simulink model "test_ffts"  (Simulink 6.2)
settings: Solver=ode45  StartTime=0.0  StopTime=300  RelTol=1e-3
undefined symbols (not defined in the file or in its folder): now
libraries: xbsIndex_r3 x1135, fft_library x1, simulink x1
(part 1 of 15)
settings Model: LastModifiedBy=mdexter
settings DebuggingCC: SolverPrmCheckMsg=warning

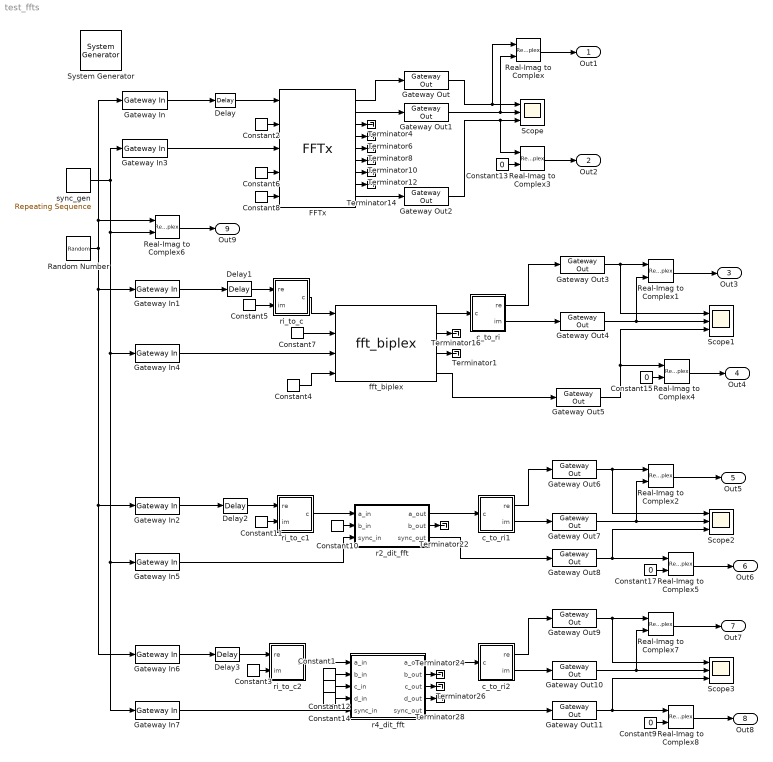
== system test_ffts ==
  " System Generator" : xbsIndex_r3/ System Generator  Tag=genX  xilinxfamily=Virtex2  part=xc2v1000  speed=-4  package=bg575  synthesis_tool=XST  directory=./netlist  testbench=off  simulink_period=1  sysclk_period=100  incr_netlist=off  trim_vbits=Everywhere in SubSystem  dbl_ovrd=According to Block Masks  core_generation=According to Block Masks  run_coregen=off  deprecated_control=off  eval_field=0
      settings: AttributesFormatString=System\nGenerator
  Constant{1,10,12,14} (4 alike) : xbsIndex_r3/Constant  const=0  equ=P=C  arith_type=Unsigned  n_bits=16  bin_pt=0  opselect=C  inp2=PCIN>>17  opr=+  inp1=P  carry=CIN  iostate=0  explicit_period=on  period=1  dbl_ovrd=off
  Constant11 : xbsIndex_r3/Constant  const=0  equ=P=C  arith_type=Unsigned  n_bits=8  bin_pt=7  opselect=C  inp2=PCIN>>17  opr=+  inp1=P  carry=CIN  iostate=0  explicit_period=on  period=1  dbl_ovrd=off
  Constant{9,13,15,17} (4 alike) : Constant  Value=0
  Constant2 : xbsIndex_r3/Constant  const=0  equ=P=C  arith_type="Signed  (2's comp)"  n_bits=8  bin_pt=7  opselect=C  inp2=PCIN>>17  opr=+  inp1=P  carry=CIN  iostate=0  explicit_period=on  period=1  dbl_ovrd=off
  Constant3 : xbsIndex_r3/Constant  const=0  equ=P=C  arith_type=Unsigned  n_bits=8  bin_pt=7  opselect=C  inp2=PCIN>>17  opr=+  inp1=P  carry=CIN  iostate=0  explicit_period=on  period=1  dbl_ovrd=off
  Constant4 : xbsIndex_r3/Constant  const=0  equ=P=C  arith_type=Unsigned  n_bits=6  bin_pt=0  opselect=C  inp2=PCIN>>17  opr=+  inp1=P  carry=CIN  iostate=0  explicit_period=on  period=1  dbl_ovrd=off
  Constant5 : xbsIndex_r3/Constant  const=0  equ=P=C  arith_type=Unsigned  n_bits=18  bin_pt=0  opselect=C  inp2=PCIN>>17  opr=+  inp1=P  carry=CIN  iostate=0  explicit_period=on  period=1  dbl_ovrd=off
  Constant6 : xbsIndex_r3/Constant  const=1  equ=P=C  arith_type=Boolean  n_bits=1  bin_pt=0  opselect=C  inp2=PCIN>>17  opr=+  inp1=P  carry=CIN  iostate=0  explicit_period=on  period=1  dbl_ovrd=off
  Constant7 : xbsIndex_r3/Constant  const=0  equ=P=C  arith_type=Unsigned  n_bits=36  bin_pt=0  opselect=C  inp2=PCIN>>17  opr=+  inp1=P  carry=CIN  iostate=0  explicit_period=on  period=1  dbl_ovrd=off
  Constant8 : xbsIndex_r3/Constant  const=1  equ=P=C  arith_type=Boolean  n_bits=1  bin_pt=0  opselect=C  inp2=PCIN>>17  opr=+  inp1=P  carry=CIN  iostate=0  explicit_period=on  period=1  dbl_ovrd=off
  Delay : xbsIndex_r3/Delay  latency=4  reg_retiming=off  explicit_period=off  period=1  en=off  accept_only_valid=off  init_zero=on  dbl_ovrd=off  show_param=off
      settings: xl_area=[0, 0, 0, 0, 0, 0, 0]
  Delay1 : xbsIndex_r3/Delay  latency=1  reg_retiming=off  explicit_period=off  period=1  en=off  accept_only_valid=off  init_zero=on  dbl_ovrd=off  show_param=off
      settings: xl_area=[0, 0, 0, 0, 0, 0, 0]
  Delay2 : xbsIndex_r3/Delay  latency=1  reg_retiming=off  explicit_period=off  period=1  en=off  accept_only_valid=off  init_zero=on  dbl_ovrd=off  show_param=off
      settings: xl_area=[0, 0, 0, 0, 0, 0, 0]
  Delay3 : xbsIndex_r3/Delay  latency=1  reg_retiming=off  explicit_period=off  period=1  en=off  accept_only_valid=off  init_zero=on  dbl_ovrd=off  show_param=off
      settings: xl_area=[0, 0, 0, 0, 0, 0, 0]
  FFTx : xbsIndex_r3/FFTx  arch=Pipelined Streaming I/O  npts=64  scaling=Unscaled  rounding=Convergent Rounding  tf_width=8  op_order=Natural Order  twiddle_mem_type=Block RAM  data_mem_type=Block RAM  num_bram_stages=0  explicit_period=off  period=-1  use_dsp48=off  en_n=off  has_ovflo=off  rst=off  en=off  dbl_ovrd=off  show_param=on  gen_core=off
      settings: xl_area=[0, 0, 0, 0, 0, 0, 0]
  Gateway In : xbsIndex_r3/Gateway In  arith_type="Signed  (2's comp)"  n_bits=8  bin_pt=7  quantization="Round  (unbiased: +/- Inf)"  overflow=Wrap  period=1  timing_constraint=None  locs_specified=off  LOCs={}  needs_fixed_name=off  dbl_ovrd=off  show_param=off
      settings: xl_area=[0, 0, 0, 0, 0, 0, 0]
  Gateway In1 : xbsIndex_r3/Gateway In  arith_type="Signed  (2's comp)"  n_bits=18  bin_pt=14  quantization="Round  (unbiased: +/- Inf)"  overflow=Wrap  period=1  timing_constraint=None  locs_specified=off  LOCs={}  needs_fixed_name=off  dbl_ovrd=off  show_param=off
      settings: xl_area=[0, 0, 0, 0, 0, 0, 0]
  Gateway In2 : xbsIndex_r3/Gateway In  arith_type="Signed  (2's comp)"  n_bits=8  bin_pt=7  quantization="Round  (unbiased: +/- Inf)"  overflow=Wrap  period=1  timing_constraint=None  locs_specified=off  LOCs={}  needs_fixed_name=off  dbl_ovrd=off  show_param=off
      settings: xl_area=[0, 0, 0, 0, 0, 0, 0]
  Gateway In{3..5,7} (4 alike) : xbsIndex_r3/Gateway In  arith_type=Boolean  n_bits=8  bin_pt=7  quantization=Truncate  overflow=Wrap  period=1  timing_constraint=None  locs_specified=off  LOCs={}  needs_fixed_name=off  dbl_ovrd=off  show_param=off
      settings: xl_area=[0, 0, 0, 0, 0, 0, 0]
  Gateway In6 : xbsIndex_r3/Gateway In  arith_type="Signed  (2's comp)"  n_bits=8  bin_pt=7  quantization="Round  (unbiased: +/- Inf)"  overflow=Wrap  period=1  timing_constraint=None  locs_specified=off  LOCs={}  needs_fixed_name=off  dbl_ovrd=off  show_param=off
      settings: xl_area=[0, 0, 0, 0, 0, 0, 0]
  Gateway Out{,1..11} (12 alike) : xbsIndex_r3/Gateway Out  output_type=Double  nbits=8  bin_pt=6  arith_type=Boolean  quantization=Truncate  overflow=Wrap  hdl_port=on  timing_constraint=None  locs_specified=off  LOCs={}  needs_fixed_name=off  show_param=off
      settings: xl_area=[0, 0, 0, 0, 0, 0, 0]
  Random Number : RandomNumber  Variance=.3^2  Seed=floor(100*(now-floor(now)))  SampleTime=1
  Real-Imag to Complex{,1..8} (9 alike) : RealImagToComplex
  Scope{,1..3} (4 alike) : Scope  NumInputPorts=3
      Scope settings: YMin=-5~-5~-5  YMax=5~5~5
      Scope1 settings: YMin=-5~-5~-5  YMax=5~5~5
      Scope2 settings: YMin=-5~-5~-5  YMax=5~5~5  SaveName=ScopeData2
      Scope3 settings: YMin=-5~-5~-5  YMax=5~5~5  SaveName=ScopeData3
  Terminator{1,4,6,8,10,12,14,16,22,24,26,28} (12 alike) : Terminator
  c_to_ri : Subsystem  mask(Complex to Real-Imag){n_bits=18, bin_pt=14}
      mask prompts: n_bits "Bit Width"; bin_pt "Binary Point"
      mask help: Outputs real and imaginary components of a complex input.
      mask init:
      | c_to_ri_init(gcb,n_bits,bin_pt);
      settings: AttributesFormatString=%<n_bits>_%<bin_pt> r/i
      mask Help:
      | <pre>
      | Description::
      | 
      | Outputs real and imaginary components of a complex input.
      | Useful for simplifying interconnects.
      | See also: Real-Imag to Complex (ri_to_c)
      | 
      | Mask Parameters::
      | 
      | Bit Width (n_bits): Specifies the width of the real/imaginary components.
      | Assumed equal for both components.
      | 
      | Binary Point (bin_pt): Specifies the binary point location in the real/imaginary components.
      | Assumed equal for both components.
      | </pre>
  c_to_ri1 : Subsystem  mask(Complex to Real-Imag){n_bits=14, bin_pt=7}
      mask prompts: n_bits "Bit Width"; bin_pt "Binary Point"
      mask help: Outputs real and imaginary components of a complex input.
      mask init:
      | c_to_ri_init(gcb,n_bits,bin_pt);
      settings: AttributesFormatString=14_7 r/i
      mask Help:
      | <pre>
      | Description::
      | 
      | Outputs real and imaginary components of a complex input.
      | Useful for simplifying interconnects.
      | See also: Real-Imag to Complex (ri_to_c)
      | 
      | Mask Parameters::
      | 
      | Bit Width (n_bits): Specifies the width of the real/imaginary components.
      | Assumed equal for both components.
      | 
      | Binary Point (bin_pt): Specifies the binary point location in the real/imaginary components.
      | Assumed equal for both components.
      | </pre>
  c_to_ri2 : Subsystem  mask(Complex to Real-Imag){n_bits=14, bin_pt=7}
      mask prompts: n_bits "Bit Width"; bin_pt "Binary Point"
      mask help: Outputs real and imaginary components of a complex input.
      mask init:
      | c_to_ri_init(gcb,n_bits,bin_pt);
      settings: AttributesFormatString=%<n_bits>_%<bin_pt> r/i
      mask Help:
      | <pre>
      | Description::
      | 
      | Outputs real and imaginary components of a complex input.
      | Useful for simplifying interconnects.
      | See also: Real-Imag to Complex (ri_to_c)
      | 
      | Mask Parameters::
      | 
      | Bit Width (n_bits): Specifies the width of the real/imaginary components.
      | Assumed equal for both components.
      | 
      | Binary Point (bin_pt): Specifies the binary point location in the real/imaginary components.
      | Assumed equal for both components.
      | </pre>
  fft_biplex : fft_library/fft_biplex  FFTSize=6  BitWidth=18  quantization="Round  (unbiased: Even Values)"  overflow=Saturate  add_latency=1  mult_latency=3  bram_latency=1
      link override biplex_core/fft_stage_1/sync_delay_x/Constant: equ=P=C
      link override biplex_core/fft_stage_1/sync_delay_x/Constant1: equ=P=C
      link override biplex_core/fft_stage_1/sync_delay_x/Constant2: equ=P=C
      link override biplex_core/fft_stage_1/sync_delay_x/Constant3: equ=P=C
      link override biplex_core/fft_stage_2/sync_delay_x/Constant: equ=P=C
      link override biplex_core/fft_stage_2/sync_delay_x/Constant1: equ=P=C
      link override biplex_core/fft_stage_2/sync_delay_x/Constant2: equ=P=C
      link override biplex_core/fft_stage_2/sync_delay_x/Constant3: equ=P=C
      link override biplex_core/fft_stage_3/sync_delay_x/Constant: equ=P=C
      link override biplex_core/fft_stage_3/sync_delay_x/Constant1: equ=P=C
      link override biplex_core/fft_stage_3/sync_delay_x/Constant2: equ=P=C
      link override biplex_core/fft_stage_3/sync_delay_x/Constant3: equ=P=C
      link override biplex_core/fft_stage_4/sync_delay_x/Constant: equ=P=C
      link override biplex_core/fft_stage_4/sync_delay_x/Constant1: equ=P=C
      link override biplex_core/fft_stage_4/sync_delay_x/Constant2: equ=P=C
      link override biplex_core/fft_stage_4/sync_delay_x/Constant3: equ=P=C
      link override biplex_core/fft_stage_5/sync_delay_x/Constant: equ=P=C
      link override biplex_core/fft_stage_5/sync_delay_x/Constant1: equ=P=C
      link override biplex_core/fft_stage_5/sync_delay_x/Constant2: equ=P=C
      link override biplex_core/fft_stage_5/sync_delay_x/Constant3: equ=P=C
      link override biplex_core/fft_stage_6/sync_delay_x/Constant: equ=P=C
      link override biplex_core/fft_stage_6/sync_delay_x/Constant1: equ=P=C
      link override biplex_core/fft_stage_6/sync_delay_x/Constant2: equ=P=C
      link override biplex_core/fft_stage_6/sync_delay_x/Constant3: equ=P=C
      link override biplex_cplx_unscrambler/delay_bram1/Constant2: equ=P=C
      link override biplex_cplx_unscrambler/reorder/Constant: equ=P=C
      link override biplex_cplx_unscrambler/reorder/sync_delay/Constant: equ=P=C
      link override biplex_cplx_unscrambler/reorder/sync_delay/Constant1: equ=P=C
      link override biplex_cplx_unscrambler/reorder/sync_delay/Constant2: equ=P=C
      link override biplex_cplx_unscrambler/reorder/sync_delay/Constant3: equ=P=C
      link override biplex_cplx_unscrambler/reorder1/Constant: equ=P=C
      link override biplex_cplx_unscrambler/reorder1/sync_delay/Constant: equ=P=C
      link override biplex_cplx_unscrambler/reorder1/sync_delay/Constant1: equ=P=C
      link override biplex_cplx_unscrambler/reorder1/sync_delay/Constant2: equ=P=C
      link override biplex_cplx_unscrambler/reorder1/sync_delay/Constant3: equ=P=C
      link override biplex_cplx_unscrambler/sync_delay/Constant: equ=P=C
      link override biplex_cplx_unscrambler/sync_delay/Constant1: equ=P=C
      link override biplex_cplx_unscrambler/sync_delay/Constant2: equ=P=C
      link override biplex_cplx_unscrambler/sync_delay/Constant3: equ=P=C
  r2_dit_fft : Subsystem  AncestorBlock=newfft_library/FFT/r2_dit_fft  mask(Biplex Radix-2 DIT FFT){n_stages=6, n_bits=8, bin_pt=7, shifts=[0], commutator_bram=0, twiddle_bram=0, n_bits_w=9, mult_latency=3, add_latency=1, commute_output=Yes (BRAM), output_order=Normal, show_sbo=on, munge_submasks=DumbDown}
      mask prompts: n_stages "Total Stages"; n_bits "Number of Bits In"; bin_pt "Binary Point In"; shifts "Shifting Schedule"; commutator_bram "Number of Stages Using BRAM for Biplex Commutators (i.e. delays)"; twiddle_bram "Number of Stages Using BRAM for Twiddle Coefficients"; n_bits_w "Twiddle Coefficient Bitwidth"; mult_latency "Multiplier Latency"; add_latency "Adder Latency"; commute_output "Commute Output"; output_order "Output Order"; show_sbo "Show Sub-Block Options"; munge_submasks "Sub-Block Masks"
      mask help: A biplex radix-2 decimation-in-time Fast Fourier Transform.
      mask init:
      | tic
      | r2_dit_fft_init(gcb, ...
      |   n_stages, ...
      |   n_bits, ...
      |   bin_pt, ...
      |   shifts, ...
      |   commutator_bram, ...
      |   twiddle_bram, ...
      |   n_bits_w, ...
      |   mult_latency, ...
      |   add_latency, ...
      |   commute_output, ...
      |   output_order, ...
      |   lower(get_param(gcb,'munge_submasks')) );
      | disp('r2_dit_fft initialization complete.');
      | toc
      settings: AttributesFormatString=|
      | 64 points
      | 8_7 r/i in
      | 9_7 twiddles
      mask Help:
      | <pre>
      | Description::
      | 
      | A biplex radix-2 decimation-in-time Fast Fourier Transform.
      | 
      | The two inputs to the biplex FFT are independent complex signals (e.g. A and B).
      | 
      | Without an output commutator, the two outputs of the FFT are commuted such that the a_out
      | signal is really the "lower" half of A's transform followed by the "lower" half of B's
      | transform and b_out is really the "upper" half of A's transform followed by the "upper"
      | half of B's transform.
      | 
      | If it is desired to have the two halves of A's transform follow each other on the same path
      | and the two halves of B's transform follow each other on the same path, then be sure to
      | check the "Output Commutator" checkbox.  This will result in the "lower" half of A (or B)
      | followed by the "upper" half of A (or B).  Including the output commutator uses additional
      | resources.
      | 
      | If the "Normal" Ouput Order option is chosen, the output will be in normal order (though still in
      | commuted halves if no output commutator is used).  If the "Bit Reversed" Output Order" option is
      | selected, the output halves (either commuted or not) will each be in bit reversed order
      | (i.e. each half of each transform will be in bit reversed output order).   Normal output is easier
      | for humans to work with (especially for testing), but it uses additional resources.  Bit reversed
      | output is the implementation's inhernet output order so that option uses no additional resources.
      | 
      | The number of bits for each real and imaginary component grows by two through each stage.
      | If a stage's input bit width is 17 or less, three embedded multipliers will be used per complex multiply.
      | If a stage's input bit width is 18, four embedded multipliers will be used per complex multiply.
      | If a stage's input bit width exceeds 18, then substantially more embedded multipliers will be used
      | per complex multiply.  Enabling "shifting" in some (or all) stages can limit the bit growth
      | to prevent this.  See the Shifting Schedule parameter for more info.
      | 
      | Mask Parameters::
      | 
      | Total Stages (n_stages):  The number of total stages in the FFT.
      | The FFT will have 2^n_stages points.
      | 
      | Number of Bits In (n_bits): Specifies the width of the real/imaginary components of ports
      | a_in and b_in.  Assumed equal for both components.  The output bit width will be
      | n_bits+n_stages (assuming sum(shifts)==0).
      | 
      | Binary Point In (bin_pt): Specifies the binary point position of the real/imaginary
      | components of ports a_in and b_in.  Assumed equal for both components.
      | 
      | Shifting Schedule (shifts): A vector specifying how many bits to shift by at each stage.
      | Missing values are assumed to be zero; extra values are ignored.
      | 
      | Number of Stages Using BRAM for Biplex Commutators (commutator_bram): Number of stages
      | that will use BRAM for commutator memory.  Remaining stages will use SLR16 elements (slices).
      | 
      | Number of Stages Using BRAM for Twiddle Coefficients (twiddle_bram): Number of stages that
      | will use BRAM for twiddle coeeficient storage.  Remaining stages will use distributed memory
      | (slices).
      | 
      | Twiddle Coefficient Bitwidth (n_bits_w): Specifies the width of the real/imaginary
      | components of the twiddle coefficients.  Assumed equal for both components.
      | 
      | Multiplier Latency (mult_latency): Latency to use for the underlying real multipliers.
      | 
      | Adder Latency (add_latency): Latency to use for the underlying real adders.
      | 
      | Commute Output (commute_output): Popup options for an output commutator.  See decription
      | above for details on the output commutator.  Choices are:
      |     "No" - No output commutator
      |     "Yes (SLR16)" - Include output commutator using SLR16 elements
      |     "Yes (BRAM)" - Include output commutator using BRAM
      | 
      | Output Order (output_order): Popup options for selecting the output order.  See description
      | above for details on the output order.  Choices are:
      |     "Bit Reversed" - Output each half of each transform in bit reversed order.
      |     "Normal" - Output each half of each transform in normal order.
      | </pre>
      mask StyleString: edit,edit,edit,edit,edit,edit,edit,edit,edit,popup(No|Yes (SLR16)|Yes (BRAM)),popup(Bit Reversed|Normal),checkbox,popup(Keep|DumbDown|Unmask)
      mask CallbackString:
      | |||||||||||mvs=get_param(gcb,'MaskVisibilityString');
      | if strcmp(get_param(gcb,'show_sbo'),'on')
      |   onoff='on';
      | else
      |   onoff='off';
      | end
      | mvs=regexprep(mvs,'o[nf]*$',onoff);
      | set_param(gcb,'MaskVisibilityString',mvs);
      | |mvs=get_param(gcb,'MaskVisibilityString');
      | if strcmp(get_param(gcb,'show_sbo'),'on')
      |   onoff='on';
      | else
      |   onoff='off';
      | end
      | mvs=regexprep(mvs,'o[nf]*$',onoff);
      | set_param(gcb,'MaskVisibilityString',mvs);
  r4_dit_fft : Subsystem  AncestorBlock=newfft_library/FFT/r4_dit_fft  mask(Quadplex Radix-4 DIT FFT){n_stages=3, n_bits=8, bin_pt=7, shifts=[0], commutator_bram=0, twiddle_bram=0, n_bits_w=9, mult_latency=3, add_latency=1, commute_output=Yes (SLR16), output_order=Normal, show_sbo=on, munge_submasks=DumbDown}
      mask prompts: n_stages "Total Stages"; n_bits "Number of Bits In"; bin_pt "Binary Point In"; shifts "Shifting Schedule"; commutator_bram "Number of Stages Using BRAM for Biplex Commutators (i.e. delays)"; twiddle_bram "Number of Stages Using BRAM for Twiddle Coefficients"; n_bits_w "Twiddle Coefficient Bitwidth"; mult_latency "Multiplier Latency"; add_latency "Adder Latency"; commute_output "Commute Output"; output_order "Output Order"; show_sbo "Show Sub-Block Options"; munge_submasks "Sub-Block Masks"
      mask help: A quadplex radix-4 decimation-in-time Fast Fourier Transform.
      mask init:
      | tic
      | r4_dit_fft_init(gcb, ...
      |   n_stages, ...
      |   n_bits, ...
      |   bin_pt, ...
      |   shifts, ...
      |   commutator_bram, ...
      |   twiddle_bram, ...
      |   n_bits_w, ...
      |   mult_latency, ...
      |   add_latency, ...
      |   commute_output, ...
      |   output_order, ...
      |   lower(get_param(gcb,'munge_submasks')) );
      | disp('r4_dit_fft initialization complete.');
      | toc
      settings: AttributesFormatString=|
      | 64 points
      | 8_7 r/i in
      | 9_7 twiddles
      mask Help:
      | <pre>
      | Description::
      | 
      | A quadplex radix-4 decimation-in-time Fast Fourier Transform.
      | 
      | The four inputs to the quadplex FFT are independent complex signals (e.g. A, B, C, D).
      | 
      | Without an output commutator, the four outputs of the FFT are commuted such that the
      | a_out signal is really the first quarter of A's transform followed by the first quarter of B's
      | transform, the first quarter of C's transform and the first quarter of D's transform.
      | b_out is really the seconds quarter of A's transform followed by the second quarter of
      | B's transform and so on for the rest of b_out as well as c_out and d_out.
      | 
      | If it is desired to have the four quarters of A's transform follow each other on the
      | same path (and so on for the transforms of B, C, and D), then be sure to check the
      | "Output Commutator" checkbox.  This will result in the four quarters of A's transform
      | (or B's, C's, D's) being in sequential order.  Including the output commutator uses additional
      | resources.
      | 
      | If the Normal Ouput Order option is chosen, the output will be in normal order (though still in
      | commuted quarters if no output commutator is used).  If the "Bit Reversed" Output Order"
      | option is selected, the output quarters (either commuted or not) will each be in bit reversed
      | order (i.e. each quarter of each transform will be in bit reversed output order).   Normal output
      | is easier for humans to work with (especially for testing), but it uses additional resources.
      | Bit reversed output is the implementation's inhernet output order so that option uses no
      | additional resources.
      | 
      | 
      | The number of bits for each real and imaginary component grows by two through this stage.
      | If the bit width grows to exceed 17 bits (when using three real multiplies per complex multiply;
      | 18 bits when using 4 real multiplies per complex multiply), then subsequent stages will
      | comsume more FPGA resources.  A future version will provide an option to limit bit growth.
      | 
      | The number of bits for each real and imaginary component grows by two through each stage.
      | If a stage's input bit width is 17 or less, three embedded multipliers will be used per complex multiply.
      | If a stage's input bit width is 18, four embedded multipliers will be used per complex multiply.
      | If a stage's input bit width exceeds 18, then substantially more embedded multipliers will be used
      | per complex multiply.  Enabling "shifting" in some (or all) stages can limit the bit growth
      | to prevent this.  See the Shifting Schedule parameter for more info.
      | 
      | 
      | Mask Parameters::
      | 
      | Total Stages (n_stages):  The number of total stages in the FFT.
      | The FFT will have 4^n_stages points.
      | 
      | Number of Bits In (n_bits): Specifies the width of the real/imaginary components of ports
      | a_in and b_in.  Assumed equal for both components.  The output bit width will be
      | n_bits+2*n_stages (assuming sum(shifts)==0).
      | 
      | Binary Point In/Out (bin_pt): Specifies the binary point position of the real/imaginary
      | components of ports a_in, b_in, c_in, and d_in.  Assumed equal for both components.
      | 
      | Shifting Schedule (shifts): A vector specifying how many bits to shift by at each stage.
      | Missing values are assumed to be zero; extra values are ignored.
      | 
      | Number of Stages Using BRAM for Biplex Commutators (commutator_bram): Number of stages
      | that will use BRAM for commutator memory.  Remaining stages will use SLR16 elements (slices).
      | 
      | Number of Stages Using BRAM for Twiddle Coefficients (twiddle_bram): Number of stages that
      | will use BRAM for twiddle coeeficient storage.  Remaining stages will use distributed memory
      | (slices).
      | 
      | Twiddle Coefficient Bitwidth (n_bits_w): Specifies the width of the real/imaginary
      | components of the twiddle coefficients.  Assumed equal for both components.
      | 
      | Multiplier Latency (mult_latency): Latency to use for the underlying real multipliers.
      | 
      | Adder Latency (add_latency): Latency to use for the underlying real adders.
      | 
      | Commute Output (commute_output): Popup options for an output commutator.  See decription
      | above for details on the output commutator.  Choices are:
      |     "No" - No output commutator
      |     "Yes (SLR16)" - Include output commutator using SLR16 elements
      |     "Yes (BRAM)" - Include output commutator using BRAM
      | 
      | Output Order (output_order): Popup options for selecting the output order.  See description
      | above for details on the output order.  Choices are:
      |     "Bit Reversed" - Output each half of each transform in bit reversed order.
      |     "Normal" - Output each half of each transform in normal order.
      | </pre>
      mask StyleString: edit,edit,edit,edit,edit,edit,edit,edit,edit,popup(No|Yes (SLR16)|Yes (BRAM)),popup(Bit Reversed|Normal),checkbox,popup(Keep|DumbDown|Unmask)
      mask CallbackString:
      | |||||||||||mvs=get_param(gcb,'MaskVisibilityString');
      | if strcmp(get_param(gcb,'show_sbo'),'on')
      |   onoff='on';
      | else
      |   onoff='off';
      | end
      | mvs=regexprep(mvs,'o[nf]*$',onoff);
      | set_param(gcb,'MaskVisibilityString',mvs);
      | |
  ri_to_c : Subsystem  mask(Real-Imag to Complex){}
      mask help: Concatenates real and imaginary inputs into a complex output.
      mask init:
      | ri_to_c_init(gcb);
      mask Help:
      | <pre>
      | Description::
      | 
      | Concatenates a real and imaginary input into a complex output.
      | Useful for simplifying interconnects.
      | See also: Complex to Real-Imag (c_to_ri)
      | 
      | Mask Parameters::
      | 
      | (N/A)
      | </pre>
  ri_to_c1 : Subsystem  mask(Real-Imag to Complex){}
      mask help: Concatenates real and imaginary inputs into a complex output.
      mask init:
      | ri_to_c_init(gcb);
      mask Help:
      | <pre>
      | Description::
      | 
      | Concatenates a real and imaginary input into a complex output.
      | Useful for simplifying interconnects.
      | See also: Complex to Real-Imag (c_to_ri)
      | 
      | Mask Parameters::
      | 
      | (N/A)
      | </pre>
  ri_to_c2 : Subsystem  mask(Real-Imag to Complex){}
      mask help: Concatenates real and imaginary inputs into a complex output.
      mask init:
      | ri_to_c_init(gcb);
      mask Help:
      | <pre>
      | Description::
      | 
      | Concatenates a real and imaginary input into a complex output.
      | Useful for simplifying interconnects.
      | See also: Complex to Real-Imag (c_to_ri)
      | 
      | Mask Parameters::
      | 
      | (N/A)
      | </pre>
  sync_gen : simulink/Sources/Repeating Sequence  rep_seq_t=[0:64]  rep_seq_y=[1 zeros(1,63) 1]
  Out1 : Outport
  Out2 : Outport  Port=2
  Out3 : Outport  Port=3
  Out4 : Outport  Port=4
  Out5 : Outport  Port=5
  Out6 : Outport  Port=6
  Out7 : Outport  Port=7
  Out8 : Outport  Port=8
  Out9 : Outport  Port=9
  wires:
  Constant2/1 -> FFTx/2
  Constant6/1 -> FFTx/4
  Constant8/1 -> FFTx/5
  FFTx/2 -> Gateway Out1/1
  FFTx/3 -> Terminator4/1
  FFTx/4 -> Terminator6/1
  FFTx/5 -> Terminator8/1
  FFTx/6 -> Terminator10/1
  FFTx/7 -> Terminator12/1
  FFTx/8 -> Terminator14/1
  FFTx/9 -> Gateway Out2/1
  Gateway In3/1 -> FFTx/3
  Delay/1 -> FFTx/1
  Gateway In/1 -> Delay/1
  Gateway Out1/1 -> Real-Imag to Complex/2, Scope/2
  Gateway Out2/1 -> Scope/3, Real-Imag to Complex3/1
  Random Number/1 -> Gateway In1/1, Gateway In2/1, Gateway In6/1, Gateway In/1, Real-Imag to Complex6/1
  Gateway In1/1 -> Delay1/1
  Gateway Out3/1 -> Scope1/1, Real-Imag to Complex1/1
  Gateway Out4/1 -> Scope1/2, Real-Imag to Complex1/2
  Gateway Out5/1 -> Scope1/3, Real-Imag to Complex4/1
  fft_biplex/4 -> Gateway Out5/1
  fft_biplex/2 -> Terminator16/1
  ri_to_c/1(c) -> fft_biplex/1
  Constant5/1 -> ri_to_c/2(im)
  Gateway In5/1 -> r2_dit_fft/3(sync_in)
  Gateway In2/1 -> Delay2/1
  Gateway Out6/1 -> Real-Imag to Complex2/1, Scope2/1
  Gateway Out7/1 -> Scope2/2, Real-Imag to Complex2/2
  Gateway Out8/1 -> Scope2/3, Real-Imag to Complex5/1
  r2_dit_fft/3(sync_out) -> Gateway Out8/1
  Constant10/1 -> r2_dit_fft/2(b_in)
  r2_dit_fft/1(a_out) -> c_to_ri1/1(c)
  c_to_ri/2(im) -> Gateway Out4/1
  r2_dit_fft/2(b_out) -> Terminator22/1
  ri_to_c1/1(c) -> r2_dit_fft/1(a_in)
  Constant11/1 -> ri_to_c1/2(im)
  Constant4/1 -> fft_biplex/4
  Constant7/1 -> fft_biplex/2
  fft_biplex/1 -> c_to_ri/1(c)
  sync_gen/1 -> Gateway In3/1, Gateway In4/1, Gateway In5/1, Gateway In7/1, Real-Imag to Complex6/2
  Gateway In4/1 -> fft_biplex/3
  Delay1/1 -> ri_to_c/1(re)
  Delay2/1 -> ri_to_c1/1(re)
  fft_biplex/3 -> Terminator1/1
  Gateway Out/1 -> Real-Imag to Complex/1, Scope/1
  FFTx/1 -> Gateway Out/1
  Real-Imag to Complex/1 -> Out1/1
  c_to_ri/1(re) -> Gateway Out3/1
  Real-Imag to Complex1/1 -> Out3/1
  c_to_ri1/1(re) -> Gateway Out6/1
  c_to_ri1/2(im) -> Gateway Out7/1
  Real-Imag to Complex2/1 -> Out5/1
  Real-Imag to Complex3/1 -> Out2/1
  Real-Imag to Complex4/1 -> Out4/1
  Real-Imag to Complex5/1 -> Out6/1
  Constant13/1 -> Real-Imag to Complex3/2
  Constant15/1 -> Real-Imag to Complex4/2
  Constant17/1 -> Real-Imag to Complex5/2
  Real-Imag to Complex6/1 -> Out9/1
  Gateway In7/1 -> r4_dit_fft/5(sync_in)
  Gateway In6/1 -> Delay3/1
  Gateway Out9/1 -> Real-Imag to Complex7/1, Scope3/1
  Gateway Out10/1 -> Scope3/2, Real-Imag to Complex7/2
  Gateway Out11/1 -> Scope3/3, Real-Imag to Complex8/1
  r4_dit_fft/5(sync_out) -> Gateway Out11/1
  Constant1/1 -> r4_dit_fft/2(b_in)
  r4_dit_fft/1(a_out) -> c_to_ri2/1(c)
  ri_to_c2/1(c) -> r4_dit_fft/1(a_in)
  Constant3/1 -> ri_to_c2/2(im)
  Delay3/1 -> ri_to_c2/1(re)
  c_to_ri2/1(re) -> Gateway Out9/1
  c_to_ri2/2(im) -> Gateway Out10/1
  Real-Imag to Complex7/1 -> Out7/1
  Real-Imag to Complex8/1 -> Out8/1
  Constant9/1 -> Real-Imag to Complex8/2
  Constant12/1 -> r4_dit_fft/3(c_in)
  Constant14/1 -> r4_dit_fft/4(d_in)
  r4_dit_fft/2(b_out) -> Terminator24/1
  r4_dit_fft/3(c_out) -> Terminator26/1
  r4_dit_fft/4(d_out) -> Terminator28/1

== system test_ffts/c_to_ri ==
  c : Inport  Port=1  LatchInput=off
  force_im : xbsIndex_r3/Reinterpret  force_arith_type=on  arith_type="Signed  (2's comp)"  force_bin_pt=on  bin_pt=14  force_valid=on
  force_re : xbsIndex_r3/Reinterpret  force_arith_type=on  arith_type="Signed  (2's comp)"  force_bin_pt=on  bin_pt=14  force_valid=on
  slice_im : xbsIndex_r3/Slice  mode=Lower Bit Location + Width  nbits=18  bit1=0  base1=MSB of Input  bit0=0  base0=LSB of Input  boolean_output=off  explicit_period=off  period=1  dbl_ovrd=off
  slice_re : xbsIndex_r3/Slice  mode=Upper Bit Location + Width  nbits=18  bit1=0  base1=MSB of Input  bit0=0  base0=LSB of Input  boolean_output=off  explicit_period=off  period=1  dbl_ovrd=off
  re : Outport
  im : Outport  Port=2
  wires:
  slice_re/1 -> force_re/1
  slice_im/1 -> force_im/1
  force_re/1 -> re/1
  force_im/1 -> im/1
  c/1 -> slice_re/1, slice_im/1

== system test_ffts/c_to_ri1 ==
  c : Inport  Port=1  LatchInput=off
  force_im : xbsIndex_r3/Reinterpret  force_arith_type=on  arith_type="Signed  (2's comp)"  force_bin_pt=on  bin_pt=7  force_valid=on
  force_re : xbsIndex_r3/Reinterpret  force_arith_type=on  arith_type="Signed  (2's comp)"  force_bin_pt=on  bin_pt=7  force_valid=on
  slice_im : xbsIndex_r3/Slice  mode=Lower Bit Location + Width  nbits=14  bit1=0  base1=MSB of Input  bit0=0  base0=LSB of Input  boolean_output=off  explicit_period=off  period=1  dbl_ovrd=off
  slice_re : xbsIndex_r3/Slice  mode=Upper Bit Location + Width  nbits=14  bit1=0  base1=MSB of Input  bit0=0  base0=LSB of Input  boolean_output=off  explicit_period=off  period=1  dbl_ovrd=off
  re : Outport
  im : Outport  Port=2
  wires:
  c/1 -> slice_im/1, slice_re/1
  force_im/1 -> im/1
  force_re/1 -> re/1
  slice_im/1 -> force_im/1
  slice_re/1 -> force_re/1

== system test_ffts/c_to_ri2 ==
  c : Inport  Port=1  LatchInput=off
  force_im : xbsIndex_r3/Reinterpret  force_arith_type=on  arith_type="Signed  (2's comp)"  force_bin_pt=on  bin_pt=7  force_valid=on
  force_re : xbsIndex_r3/Reinterpret  force_arith_type=on  arith_type="Signed  (2's comp)"  force_bin_pt=on  bin_pt=7  force_valid=on
  slice_im : xbsIndex_r3/Slice  mode=Lower Bit Location + Width  nbits=14  bit1=0  base1=MSB of Input  bit0=0  base0=LSB of Input  boolean_output=off  explicit_period=off  period=1  dbl_ovrd=off
  slice_re : xbsIndex_r3/Slice  mode=Upper Bit Location + Width  nbits=14  bit1=0  base1=MSB of Input  bit0=0  base0=LSB of Input  boolean_output=off  explicit_period=off  period=1  dbl_ovrd=off
  re : Outport
  im : Outport  Port=2
  wires:
  c/1 -> slice_im/1, slice_re/1
  force_im/1 -> im/1
  force_re/1 -> re/1
  slice_im/1 -> force_im/1
  slice_re/1 -> force_re/1
